simulink model "chap8_9sim"  (R2015a)
settings: Solver=ode45  StartTime=0.0  StopTime=20  RelTol=1e-3
settings Model: Creator=zhr  LastModifiedBy=zhr

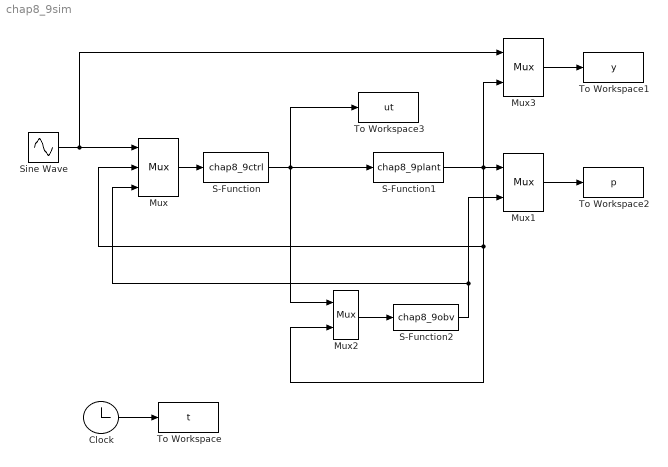
== system chap8_9sim ==
  Clock : Clock
  Mux : Mux  Inputs=3
  Mux1 : Mux  Inputs=2
  Mux2 : Mux  Inputs=2
  Mux3 : Mux  Inputs=2
  S-Function : S-Function  FunctionName=chap8_9ctrl
  S-Function1 : S-Function  FunctionName=chap8_9plant
  S-Function2 : S-Function  FunctionName=chap8_9obv
  Sine Wave : Sin  Amplitude=150  Frequency=0.5  SampleTime=0
  To Workspace : ToWorkspace  VariableName=t  SampleTime=-1
  To Workspace1 : ToWorkspace  VariableName=y  SampleTime=-1
  To Workspace2 : ToWorkspace  VariableName=p  SampleTime=-1
  To Workspace3 : ToWorkspace  VariableName=ut  SampleTime=-1
  wires:
  Clock/1 -> To Workspace/1
  Sine Wave/1 -> Mux3/1, Mux/1
  Mux/1 -> S-Function/1
  S-Function/1 -> To Workspace3/1, S-Function1/1, Mux2/1
  S-Function1/1 -> Mux2/2, Mux/2, Mux3/2, Mux1/1
  S-Function2/1 -> Mux1/2, Mux/3
  Mux2/1 -> S-Function2/1
  Mux3/1 -> To Workspace1/1
  Mux1/1 -> To Workspace2/1
